simulink model "counter_OneWay"  (R2023b)
settings: Solver=VariableStepAuto  StartTime=0.0  StopTime=10.0  RelTol=1e-3
settings Model: Creator=Saurabh  LastModifiedBy=saura
settings DebuggingCC: UnconnectedInputMsg=warning  UnconnectedOutputMsg=warning  UnconnectedLineMsg=warning
settings ModelReferenceCC: EnableRefExpFcnMdlSchedulingChecks=on
settings RTWCC: DLArmComputeVersion=19.05

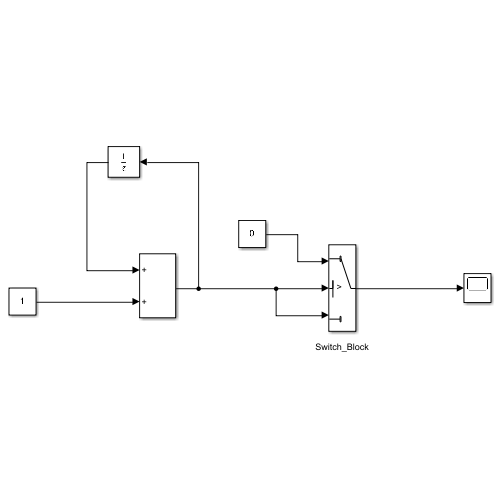
[thumbnail: Simulink's stored preview of the top-level diagram]
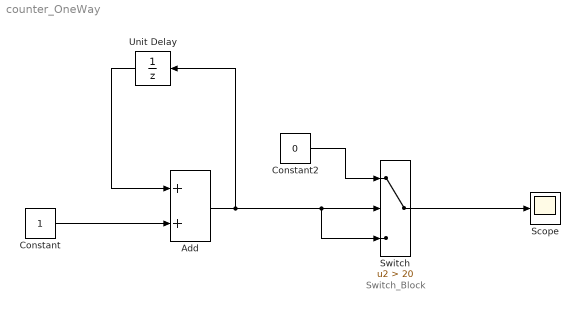
== system counter_OneWay ==
  note: Switch_Block
  Add : Sum
  Constant : Constant
  Constant2 : Constant  Value=0
  Scope : Scope
  Switch : Switch  Criteria=u2 > Threshold  Threshold=20  SaturateOnIntegerOverflow=off  InputSameDT=off
  Unit Delay : UnitDelay  SampleTime=-1  HasFrameUpgradeWarning=on
  wires:
  Constant/1 -> Add/2
  Add/1 -> Unit Delay/1, Switch/3, Switch/2
  Unit Delay/1 -> Add/1
  Switch/1 -> Scope/1
  Constant2/1 -> Switch/1
